simulink model "playback_data_4"  (R2015a)
settings: Solver=FixedStepDiscrete  SolverMode=SingleTasking  StartTime=0  StopTime=time_recorded(end)  FixedStep=sample_time  RelTol=1e-3
undefined symbols (not defined in the file): A1_notch_f1, A2_notch_f1, A_kalman_transverse, A_kalman_vertical, A_lpf_dtau, A_lpf_fourbar_angles, A_lpf_imu, A_lpf_lateral_angle, A_lpf_leg_spring, B1_lpf_dtau, B1_lpf_fourbar_angles, B1_lpf_imu, B1_lpf_lateral_angle, B1_lpf_leg_spring, B1_notch_f1, B2_lpf_dtau, B2_lpf_fourbar_angles, B2_lpf_imu, B2_lpf_lateral_angle, B2_lpf_leg_spring, B2_notch_f1, B_dx_versus_x0, B_kalman_transverse, B_kalman_vertical, backwards_K_front_of_t_row1, backwards_K_front_of_t_row2, backwards_K_sag_of_t, backwards_P_front_of_t, backwards_P_sag_of_t, C_kalman_transverse, C_kalman_vertical, com_leg_motor, com_torso, contact_threshold, control_start_time, d_ankle_to_foot, d_vertical_com, desired_com_forward_velocity, desired_com_lateral_velocity, desired_initial_leg_roll_left, desired_initial_leg_roll_right, desired_lateral_symmetry_angle, desired_standing_torso_pitch, desired_standing_torso_roll, desired_standing_z, desired_torso_pitch, desired_torso_roll, Discrete, fcut_contact, forward_dx_of_dxstar, forward_x_of_dxstar, g, gain_nodes_sea_torque, HIP_MTR_MAX_CONT_TORQUE, HIP_MTR_MAX_TORQUE, i_leg_motor, i_robot, i_torso, initial_dx_estimate, initial_dy_estimate ... (+75)
libraries: simulink x12, ctrlSharedLib x3
(part 4 of 5)

== matlab function playback_data_4/Control/Behavior Control/Primary and Lateral Behavior/Stance/LQR Feedback for Desired Frontal GRF and Roll Accleration ==
  data: hopping input; stance input; GRFy_desired output; ydy input; rolldroll input; symdsym input; zdz input; Fz input; GRF_measured input; ydy_ref input; ddroll_desired output; cost_to_go output double size=1; Roll_star input; symmetry_desired input; K_front input; P_front input; m_torso parameter; m_leg_motor parameter; lateral_offset parameter; com_torso parameter; i_torso parameter; i_leg_motor parameter; k_LQR_frontal_infinite parameter; P_LQR_frontal_infinite parameter; desired_standing_torso_roll parameter; angular_momentum output; frontal_error output
%  x_front = [y, roll, sym, dy, droll, L]; 
function [GRFy_desired, ddroll_desired, cost_to_go, angular_momentum, frontal_error]  =  ...
    LQR_Frontal(hopping, stance, ydy, rolldroll, symdsym, zdz, Fz, GRF_measured,...
           ydy_ref, Roll_star, symmetry_desired, K_front, P_front,...
           m_torso, m_leg_motor, lateral_offset, com_torso, i_torso, i_leg_motor, ...
           k_LQR_frontal_infinite, P_LQR_frontal_infinite, desired_standing_torso_roll)
    
    % Angular momentum about the pelvis in the frontal plane
    d = norm(com_torso(2:3));
    It_f = i_torso(1);
    Im_f = i_leg_motor(1);
    angular_momentum = rolldroll(2)*(m_torso*d^2 + It_f + 2*(m_leg_motor*lateral_offset^2+ Im_f)) -symdsym(2)*(m_leg_motor*lateral_offset^2+Im_f);
    feedforward_Fy = Fz*ydy_ref(1)/zdz(1);
    % feedforward_Fy = Fz*ydy(1)/zdz(1);
    frontal_state = [ydy(1); rolldroll(1); symdsym(1); ydy(2); rolldroll(2); angular_momentum];
    
    if hopping
        frontal_reference = [ydy_ref(1); Roll_star(1); symmetry_desired; ydy_ref(2); Roll_star(2); 0];
        frontal_error = frontal_state - frontal_reference;
        u = [feedforward_Fy;0]-K_front*frontal_error;
        GRFy_desired = u(1);
        ddroll_desired = u(2);
        cost_to_go = 0.5*frontal_error'*P_front*frontal_error;
        GRFy_desired = min(max(GRFy_desired, -0.5*abs(GRF_measured(3))), 0.5*abs(GRF_measured(3))); % saturate to friction cone
    else
        frontal_reference = [ydy_ref(1); desired_standing_torso_roll; symmetry_desired; ydy_ref(2); 0; 0];
        frontal_error = frontal_state - frontal_reference;
        %         frontal_error([1 4]) = 0;
        u = -k_LQR_frontal_infinite*frontal_error;
        %         u = [Fz*ydy(1)/zdz(1); 0]-k_LQR_frontal_infinite*frontal_error;
        GRFy_desired = u(1);
        ddroll_desired = u(2);
        cost_to_go = 0.5*frontal_error'*P_LQR_frontal_infinite*frontal_error;
        GRFy_desired = min(max(GRFy_desired, -0.5*abs(GRF_measured(3))), 0.5*abs(GRF_measured(3)));
    end
    
    if stance == 0
      GRFy_desired = 0;
      ddroll_desired = 0;
      cost_to_go = 0;
    end
end

== matlab function playback_data_4/Control/Behavior Control/Secondary Leg Behavior/Avoid Hitting Mechanical Limits ==
  data: back_cmd output double; front_cmd output double; dback_cmd output double; dfront_cmd output double; ddback_cmd output double; ddfront_cmd output double; back_desired input; dback_desired input; ddback_desired input; front_desired input; dfront_desired input; ddfront_desired input; min_front_bar_angle parameter; max_front_bar_angle parameter; min_back_bar_angle parameter; max_back_bar_angle parameter
%% Avoid joint limits by ensuring we don't command velocities/accelerations that would push us into them when we are close to them.
function [back_cmd, front_cmd, dback_cmd, dfront_cmd, ddback_cmd, ddfront_cmd] ...
    = AvoidFourbarLimits(back_desired,dback_desired, ddback_desired, ...
          front_desired, dfront_desired, ddfront_desired, ...
          min_front_bar_angle, max_front_bar_angle, min_back_bar_angle, max_back_bar_angle)
    [back_cmd, front_cmd, dback_cmd, dfront_cmd, ddback_cmd, ddfront_cmd] = AvoidFourbarLimits(back_desired,dback_desired, ddback_desired, front_desired, dfront_desired, ddfront_desired, min_front_bar_angle, max_front_bar_angle, min_back_bar_angle, max_back_bar_angle);
end

== matlab function playback_data_4/Control/Behavior Control/State Estimation/PositionUsingRobotGeometry ==
  data: right_left input; horizontal_com_position output; roll input; pitch input; yaw input; horizontal_com_velocity output; lateral_com_position output; lateral_com_velocity output; left_leg_sagittal_angle input; left_leg_lateral_angle input; left_leg_length input; right_leg_sagittal_angle input; right_leg_lateral_angle input; right_leg_length input; m_torso parameter; m_leg_motor parameter; m_leg parameter; com_torso parameter; com_leg_motor parameter; lateral_offset parameter; vertical_com_position output; vertical_com_velocity output; com_left_foot output; dcom_left_foot output; com_right_foot output; dcom_right_foot output; com_pelvis output; dcom_pelvis output
% Returns 2D COM relative to primary foot
function [horizontal_com_position, horizontal_com_velocity, ...
          lateral_com_position, lateral_com_velocity, ...
          vertical_com_position, vertical_com_velocity, ...
          com_left_foot, dcom_left_foot, com_right_foot, dcom_right_foot, ....
          com_pelvis, dcom_pelvis] = ...
         ComPositionUsingRobotGeometry(right_left, ...
                                    roll, pitch, yaw, ...
                                    left_leg_sagittal_angle, left_leg_lateral_angle, left_leg_length, ...
                                    right_leg_sagittal_angle, right_leg_lateral_angle, right_leg_length, ...
                                    m_torso, m_leg_motor, m_leg, com_torso, com_leg_motor, lateral_offset)
                    
    q =  [roll(1), pitch(1), yaw(1), left_leg_sagittal_angle(1), left_leg_lateral_angle(1), left_leg_length(1), right_leg_sagittal_angle(1), right_leg_lateral_angle(1), right_leg_length(1)];
    dq = [roll(2), pitch(2), yaw(2), left_leg_sagittal_angle(2), left_leg_lateral_angle(2), left_leg_length(2), right_leg_sagittal_angle(2), right_leg_lateral_angle(2), right_leg_length(2)];
                    
    [ com_pelvis, dcom_pelvis, ...
      com_left_foot, dcom_left_foot, ...
      com_right_foot, dcom_right_foot ] = ...
    ComCalculationFromRobot( q, dq, m_torso, m_leg_motor, m_leg, com_torso, com_leg_motor, lateral_offset );

    if right_left
        com_position = com_right_foot(4:6);
        com_velocity = dcom_right_foot(4:6);
    else
        com_position = com_left_foot(4:6);
        com_velocity = dcom_left_foot(4:6);
    end


    horizontal_com_position = com_position(1);
    horizontal_com_velocity = com_velocity(1);
    lateral_com_position = com_position(2);
    lateral_com_velocity = com_velocity(2);
    vertical_com_position = com_position(3);
    vertical_com_velocity = com_velocity(3);

end

== matlab function playback_data_4/Control/Behavior Control/Torque Distribution Left/Motor Torque Saturation Optimization ==
  data: x1s input; t1 output; x2s input; lambda1 parameter; lambda2 parameter; max_torque_sagittal parameter; t2 output
% Optimal leg motor torque distribution
function [t1, t2] = distribute_torque(x1s, x2s, lambda1, lambda2, max_torque_sagittal)

s = max_torque_sagittal;

% possible solutions
x1 = [                                                      x1s;
                                                            0;
                                                            s;
                                                            0;
                                                           -s;
  (lambda2*s + lambda1*x1s - lambda2*x2s)/(lambda1 + lambda2);
  (lambda1*x1s - lambda2*s + lambda2*x2s)/(lambda1 + lambda2);
  (lambda2*s + lambda1*x1s + lambda2*x2s)/(lambda1 + lambda2);
 -(lambda2*s - lambda1*x1s + lambda2*x2s)/(lambda1 + lambda2)];
 
x2 = [                                                      x2s;
                                                            s;
                                                            0;
                                                           -s;
                                                            0;
  (lambda1*s - lambda1*x1s + lambda2*x2s)/(lambda1 + lambda2);
  (lambda1*s + lambda1*x1s + lambda2*x2s)/(lambda1 + lambda2);
  (lambda1*x1s - lambda1*s + lambda2*x2s)/(lambda1 + lambda2);
 -(lambda1*s + lambda1*x1s - lambda2*x2s)/(lambda1 + lambda2)];

% test constraints
c1 = s - x1 - x2 >= 0;
c2 = s + x1 + x2 >= 0;
c3 = s - x1 + x2 >= 0;
c4 = s + x1 - x2 >= 0;
constraints = c1 & c2 & c3 & c4;

% objective function to maximize
f = -lambda1*(x1-x1s).^2-lambda2*(x2-x2s).^2;
satisfied = find(constraints);
[~,I] = max(f(satisfied));

t1 = x1(satisfied(I));
t2 = x2(satisfied(I));

== matlab function playback_data_4/Control/Behavior Control/State Estimation/Kalman Filtering/eigen values ==
  data: Z input; E output
function E = eigen(Z)
    E = real(eig(Z));
    E = sort(E);
end

== matlab function playback_data_4/Control/Behavior Control/Primary and Lateral Behavior/Flight/Generate Parabolic Foot Trajectories ==
  data: time_remaining input; est_duration input; x_star input; y_star input; x0 input; dx0 input; y0 input; dy0 input; zdz0 input; max_retract input; flight input; z_land parameter; min_f_duration parameter; X_star output size=3; Y_star output size=3; Z_star output size=3
%% Parabolic trajectory generation for x, y, and z
% est_duration: estimated flight time
% time_remaining: time until estimated touchdown
% stance: 1 if in stance, 0 otherwise
% x_star: desired x for foot to COM
% y_star: desired y for foot to COM
% x0: x position at takeoff
% y0: y position at takeoff
% zdz0: [z, dz] at takeoff
% max_retract: how high to lift z for ground clearance
% z_land: nominal z height for landing
% min_f_duration: minimum trajectory time

function [X_star, Y_star, Z_star]  =  ...
          GenerateParabolicFootTrajectory(time_remaining, est_duration,  ...
                               x_star, y_star, x0, dx0, y0, dy0, zdz0, ...
                               max_retract,  flight, z_land, min_f_duration)

if ~flight
    X_star = [0;0;0];
    Y_star = [0;0;0];
    Z_star = [0;0;0];
    return;
end
                           
% we are solving for yawed coordinates xyz of com-foot in flight and
% converting them to joint angles

% estimate z ballistically
% z = z_dz_liftoff(1) + z_dz_liftoff(2)*t_flight -g/2*t_flight^2;
% dz = z_dz_liftoff(2) - g*t_flight;
% 
% z = com_xdx_ydy_zdz(5); dz = com_xdx_ydy_zdz(6);
% time_remaining = (-dz-sqrt(max(dz^2 - 4*g/2*(z_land-z), 0) ) )/ (-g); % ballistic estimate of landing


  % plan a traj from init to desired in estimated duration. Use a
  % discontinuous initial condition if estimated duration too short.
  duration = max(est_duration, min_f_duration);
  t_r = max(min(time_remaining, duration),0);
  % sweep a parabola from x0 to x_star with dx_end = -dx0
  dx_star = dx0;
  x_star_t = x_star + dx_star*t_r + (x0-x_star-dx_star*duration)*(t_r/duration)^2;
  dx_star_t = -dx_star - 2*(x0-x_star-dx_star*duration)*(t_r/duration^2);
  ddx_star_t =  2*(x0-x_star-dx_star*duration)*(1/duration^2);
  
  % same for y
  dy_star = dy0;
  y_star_t = y_star + dy_star*t_r + (y0-y_star-dy_star*duration)*(t_r/duration)^2;
  dy_star_t = -dy_star - 2*(y0-y_star-dy_star*duration)*(t_r/duration^2);
  ddy_star_t =  2*(y0-y_star-dy_star*duration)*(1/duration^2);
  
  % Zero out velocities when out of time
  if time_remaining < 0
    dx_star_t = 0; ddx_star_t = 0;
    dy_star_t = 0; ddy_star_t = 0;
  end 
  
  % split duration into thirds.  First segment: parabola from z0 to
  % max_retract.  Second and third segments, cos to landing.
  z0 = zdz0(1);
  dt3 = duration / 3;
  z_min = z_land - max_retract;
  if t_r > 2*dt3;
    z_star_t = z_min + (z0-z_min)*((t_r-2*dt3)/dt3)^2;
    dz_star_t = -(z0-z_min)*2*(t_r-2*dt3)/dt3/dt3;
    ddz_star_t = (z0-z_min)*2/dt3^2;
  else
    z_star_t = z_land + (z_min-z_land)/2*(1-cos(t_r/(2*dt3)*pi));
    dz_star_t = -(z_min-z_land)/2*sin(t_r/(2*dt3)*pi)*pi/(2*dt3);
    ddz_star_t = (z_min-z_land)/2*cos(t_r/(2*dt3)*pi)*(pi/(2*dt3))^2;
  end
  
  % track a sinusoidal z of amplitude max_retract, finishing a half-cycle by t_end
  X_star = [x_star_t; dx_star_t; ddx_star_t];
  Y_star = [y_star_t; dy_star_t; ddy_star_t];
  Z_star = [z_star_t; dz_star_t; ddz_star_t];

== matlab function playback_data_4/Control/Behavior Control/Primary and Lateral Behavior/Stance/LQR Feedback for Desired Vertical GRF ==
  data: hopping input; stance input; zdzddz_ref input size=3; GRFz_desired output; z_state input; leg_length input; k_LQR_vertical parameter; P_LQR_vertical parameter; k_vertical_winch parameter; m_total_real parameter; g parameter; cost_to_go output double size=1; max_leg_length parameter
%% LQR for z during stance

% stance: 1 if in stance, 0 otherwise
% z_state: [z, dz] current estimate
% zdzddz_ref: reference trajectory for z position, velocity, and acceleration


% GRFz_desired: desired z GRF
% cost_to_go: remaining LQR cost

function [GRFz_desired, cost_to_go]   =  ...
               LQR_Vertical_Height(hopping, stance, zdzddz_ref, z_state, leg_length,...
                                   k_LQR_vertical, P_LQR_vertical, k_vertical_winch, m_total_real, g, max_leg_length)

    z_ref = zdzddz_ref(1:2);     
    ddz_ref = zdzddz_ref(3);
    z_error = (z_state - z_ref);
    GRFz_desired = m_total_real*(g+ddz_ref) - k_LQR_vertical*z_error;
    
    if z_ref(2) < 0
        GRFz_desired = max(50, GRFz_desired);
    elseif leg_length(1) >= max_leg_length
        GRFz_desired = 0;
    end
    
    if ~hopping
        GRFz_desired = m_total_real*g - k_vertical_winch*z_error;
        GRFz_desired = max(200, GRFz_desired);
    end
    
    cost_to_go = z_error'*P_LQR_vertical*z_error;
    
    if stance == 0
      GRFz_desired = 0;
      cost_to_go = 0;
    end
end

== matlab function playback_data_4/Control/Behavior Control/Primary and Lateral Behavior/Circular Buffer/Buffer6 ==
  data: data input; buffer output size=recorded_steps; trigger input; buffer_size input
function buffer  = buffer_data(data, trigger, buffer_size)

    persistent buffer_memory
    coder.varsize('buffer_memory',100);
    if isempty(buffer_memory)
        buffer_memory = [];
    end
    
    if trigger
        buffer_memory = [data; buffer_memory];
        if size(buffer_memory, 1) > buffer_size
            buffer_memory = buffer_memory(1:buffer_size,:);
        end
    end
    
    buffer = buffer_memory;

end

== matlab function playback_data_4/Control/Behavior Control/Primary and Lateral Behavior/Stance/COM X,Y,Z  trajectory generation ==
  data: stance input; hopping input; x_0 output size=1; y_0 output size=1; z_ref output size=1; dz_ref output size=1; ddz_ref output size=1; x_ref output size=1; dx_ref output size=1; y_ref output size=1; dy_ref output size=1; t input size=1; dx0 input; dy0 input; target_DX input; target_DY input; z_rest_new parameter; z_amplitude parameter; spring_frequency parameter; phase_0 parameter; forward_x_of_dxstar parameter; forward_dx_of_dxstar parameter; target_dx_range parameter; T_s parameter; desired_standing_z parameter
%% COM trajectory generation for stance & foot placement for flight

% Outputs:
% x_0: desired x position for COM at touchdown
% y_0: desired y position for COM at touchdown
% [z_ref, dz_ref, ddz_ref]: reference trajectory for vertical
% [x_ref, dx_ref]: reference trajectory for forward
% [y_ref, dy_ref]: reference trajectory for lateral

% Inputs:
% t: time since touchdown
% dx0: touchdown x velocity
% dy0: touchdown y velocity
% target_DX: desired x velocity at takeoff
% s_duration: nominal stance time
% z_rest_new: z height of oscillation
% target_dx_range: full range of possible x velocities in lookup table
% forward_x_of_dxstar: master lookup table for x trajectories
% T_s: tabled vector from 0 to s_duration

function [x_0, y_0,...
          z_ref, dz_ref, ddz_ref, ...
          x_ref, dx_ref, y_ref, dy_ref] ...
          = ReferenceTrajectory(stance, hopping, t, dx0, dy0, target_DX, target_DY, z_rest_new, z_amplitude, ...
            spring_frequency, phase_0, forward_x_of_dxstar, forward_dx_of_dxstar, ...
            target_dx_range, T_s,...
            desired_standing_z)
        
    % Z trajectory 
    z_ref =  z_rest_new + z_amplitude*sin(spring_frequency*t+phase_0);
    dz_ref = z_amplitude*spring_frequency*cos(spring_frequency*t+phase_0);
    ddz_ref = -z_amplitude*spring_frequency^2*sin(spring_frequency*t+phase_0);
    
    % saturate t and initial velocity to reference library
    t_sat = max( min(t, T_s(end)), 0);

    % [X, dX] trajectory from 0 to s_duration
    forward_x_given_dxstar = squeeze(interp1(target_dx_range, forward_x_of_dxstar, target_DX));
    forward_dx_given_dxstar = squeeze(interp1(target_dx_range, forward_dx_of_dxstar, target_DX));

    dx0 = max( min(dx0, max(forward_dx_given_dxstar(:,1))), min(forward_dx_given_dxstar(:,1)) );
    x_ref  = interp2(T_s, forward_dx_given_dxstar(:,1), forward_x_given_dxstar, t_sat, dx0);
    dx_ref = interp2(T_s, forward_dx_given_dxstar(:,1), forward_dx_given_dxstar, t_sat, dx0);
    x_0 = interp1(forward_dx_given_dxstar(:,1), forward_x_given_dxstar(:,1), dx0);

    % [Y, dY] trajectory from 0 to s_duration
    % Y uses same library as X
    forward_y_given_dxstar = squeeze(interp1(target_dx_range, forward_x_of_dxstar, target_DY));
    forward_dy_given_dxstar = squeeze(interp1(target_dx_range, forward_dx_of_dxstar, target_DY));

    dy0 = max( min(dy0, max(forward_dy_given_dxstar(:,1))), min(forward_dy_given_dxstar(:,1)) );
    y_ref  = interp2(T_s, forward_dy_given_dxstar(:,1), forward_y_given_dxstar, t_sat, dy0);
    dy_ref = interp2(T_s, forward_dy_given_dxstar(:,1), forward_dy_given_dxstar, t_sat, dy0);
    y_0 = interp1(forward_dy_given_dxstar(:,1), forward_y_given_dxstar(:,1), dy0);
    
    if ~hopping % Standing
        z_ref = desired_standing_z;
        dz_ref = 0;
        ddz_ref = 0;
        x_ref = 0;
        dx_ref = 0;
        y_ref = 0;
        dy_ref =0;
    elseif ~stance % Flight
        z_ref = 0;
        dz_ref = 0;
        ddz_ref = 0;
        x_ref = 0;
        dx_ref = 0;
        y_ref = 0;
        dy_ref =0;    
    end
  
end

== matlab function playback_data_4/Control/Behavior Control/Primary and Lateral Behavior/Stance/Lookup finite horizon LQR gain ==
  data: K_sag output size=[1,4]; P_sag output size=[4,4]; t_forward input; backwards_K_sag_of_t parameter; backwards_K_front_of_t_row1 parameter; backwards_K_front_of_t_row2 parameter; T_lqr parameter; stance_duration parameter; K_front output size=[2,6]; backwards_P_sag_of_t parameter; P_front output size=[6,6]; backwards_P_front_of_t parameter
%% Interpolates pregenerated finite horizon LQR gain tables 
% sagittal_state: [X, Pitch, dX, dPtich]
% frontal state: [Y; Roll; sym; dY; dRoll; angular_momentum];
function [K_sag, P_sag, K_front, P_front]  =  FiniteHorizonLQRLookup(t_forward, backwards_K_sag_of_t, backwards_K_front_of_t_row1, backwards_K_front_of_t_row2, T_lqr, stance_duration, backwards_P_sag_of_t, backwards_P_front_of_t)
  t = stance_duration - t_forward; % gains are scheduled w.r.t time until end.                                     
  t = min(max(t, min(T_lqr)), max(T_lqr));
  K_sag = interp1(T_lqr, backwards_K_sag_of_t, t);
  P_sag = squeeze(interp1(T_lqr,backwards_P_sag_of_t,t));

  % inputs for frontal LQR: backwards_K_front_of_t_row1, backwards_K_front_of_t_row2
  K_front_row1 = interp1(T_lqr, backwards_K_front_of_t_row1, t);
  K_front_row2 = interp1(T_lqr, backwards_K_front_of_t_row2, t);
  K_front = [K_front_row1; K_front_row2];
  P_front = squeeze(interp1(T_lqr,backwards_P_front_of_t,t));
end

== matlab function playback_data_4/Control/Behavior Control/Primary and Lateral Behavior/Flight/Convert COM Position to Joint Angles + Leg Length  ==
  data: hopping input; desired_leg_length output; X_star input; Y_star input; Z_star input; right_left input; com_pelvis_body input; desired_alpha output; desired_beta output; dcom_pelvis_body input; roll input; pitch input; sagittal_angle input; lateral_angle input; leg_length input; lateral_offset parameter; desired_initial_leg_roll_right parameter; desired_initial_leg_roll_left parameter; d_vertical_com parameter; desired_standing_z parameter
function [ desired_leg_length, desired_alpha, desired_beta ]  =  ...
          ConvertToJointAnglesAndLegLength(hopping, X_star, Y_star, Z_star, right_left,...
                           com_pelvis_body, dcom_pelvis_body, ...
                           roll, pitch, sagittal_angle, lateral_angle, leg_length,...
                           lateral_offset, desired_initial_leg_roll_right, desired_initial_leg_roll_left, d_vertical_com, desired_standing_z) 

    q = [roll(1), pitch(1), sagittal_angle(1), lateral_angle(1), leg_length(1)];
    dq = [roll(2), pitch(2), sagittal_angle(2), lateral_angle(2), leg_length(2)];
    [desired_alpha, desired_beta, desired_leg_length]  =  ConvertComPositionToLegAnglesAndLegLength(X_star, Y_star, Z_star, right_left, com_pelvis_body, dcom_pelvis_body, q, dq, lateral_offset);   
                       
    if ~hopping
        desired_leg_length = [desired_standing_z-d_vertical_com; 0; 0];
        desired_alpha = [pi; 0; 0];
        desired_beta = [desired_initial_leg_roll_left; 0; 0];
        if right_left
            desired_beta = [desired_initial_leg_roll_right; 0; 0];
        end
    end
    
end

== matlab function playback_data_4/Control/Behavior Control/Primary and Lateral Behavior/Circular Buffer/Buffer7 ==
  data: data input; buffer output size=recorded_steps; trigger input; buffer_size input
function buffer  = buffer_data(data, trigger, buffer_size)

    persistent buffer_memory
    coder.varsize('buffer_memory',100);
    if isempty(buffer_memory)
        buffer_memory = [];
    end
    
    if trigger
        buffer_memory = [data; buffer_memory];
        if size(buffer_memory, 1) > buffer_size
            buffer_memory = buffer_memory(1:buffer_size,:);
        end
    end
    
    buffer = buffer_memory;

end

== matlab function playback_data_4/Control/Behavior Control/Secondary Leg Behavior/Virtual Leg to Four Bar ==
  data: l_leg input; dl_leg input; ddl_leg input; phi input; dphi input; ddphi input; back output; dback output; ddback output; front output; dfront output; ddfront output
function [back, dback, ddback, front, dfront, ddfront] = VirtualLegToFourBar(l_leg, dl_leg, ddl_leg, phi, dphi, ddphi)
    [back, dback, ddback, front, dfront, ddfront] = VirtualLegToFourBar(l_leg, dl_leg, ddl_leg, phi, dphi, ddphi);
end

== matlab function playback_data_4/Control/Behavior Control/Primary and Lateral Behavior/Closed Loop Compensation/CLOSED LOOP COMPENSATION X FOR VAIRABLE SPEED ==
  data: A_cl input; epsilon input; c input; delta_s_i input; dx_star input; B_cl input; delta_ux output
function delta_ux  = closed_loop_compensation_dxstar...
         (A_cl,epsilon, c, delta_s_i, dx_star, B_cl)
% assume form of delta_s_{i+1} = A_cl*delta_s_i + epsilon +c*dx_star + B_cl*delta_ux
% where delta measures deviation from deadbeat case. solve for
% delta_ux = (-A_cl*delta_s_i-epsilon - c*dxstar)/B_cl to achieve deadbeat
delta_ux = (-A_cl*delta_s_i - epsilon - c*dx_star)/B_cl;

== matlab function playback_data_4/Control/Behavior Control/Primary and Lateral Behavior/Closed Loop Compensation/ESTIMATE CLOSED LOOP ERROR X FOR VARIABLE SPEED ==
  data: dx_land_hist input; A_cl output; delta_ux_hist input; dx_lift_hist input; dx_star_hist input; B_dx_versus_x0 parameter; W_real input; epsilon_0 output; c output; A_cl_nb output; epsilon_0_nb output; c_nb output
function [A_cl, epsilon_0, c, ...
          A_cl_nb, epsilon_0_nb, c_nb] = error_fitting_dxstar...
         (dx_land_hist, delta_ux_hist, dx_lift_hist, dx_star_hist,...
          B_dx_versus_x0, W_real)
% data_length = min([length(dx_lift_hist), filter_length]);
data_length = length(dx_lift_hist);
assert(data_length < 100);
% add fake data
fake_dx_land_err_magnitude = 0.1; fake_dx_star_magnitude = 0.1;
[fgrid_dx_land_err, fgrid_dx_star, fgrid_dx_lift_err] = ...
    meshgrid(fake_dx_land_err_magnitude*[-1 1],fake_dx_star_magnitude*[-1 1],0);
fake_data_length = numel(fgrid_dx_land_err);
fake_dx_land_err = fgrid_dx_land_err(:);
fake_dx_star = fgrid_dx_star(:);
fake_dx_lift_err = fgrid_dx_lift_err(:);
fake_delta_ux = zeros(fake_data_length,1);
% assert(fake_data_length<100);
% assert(filter_length<100);
% fake_dx_land_err = linspace(-0.1, 0.1, fake_data_length)';
% fake_dx_lift_err = zeros(fake_data_length,1);
% fake_delta_ux = zeros(fake_data_length,1);
% fake_dx_star = linspace(-0.25, 0.25, fake_data_length)';
dx_land_err = [reshape(dx_land_hist(1:data_length)-dx_star_hist(1:data_length),...
                       data_length, 1); fake_dx_land_err];
dx_lift_err = [reshape(dx_lift_hist(1:data_length)-dx_star_hist(1:data_length),...
                       data_length, 1); fake_dx_lift_err];
dx_star = [reshape(dx_star_hist(1:data_length), data_length,1); fake_dx_star];
delta_ux = [reshape(delta_ux_hist(1:data_length), data_length, 1); fake_delta_ux];
% weighted least squares
W = diag([W_real*ones(1,data_length), ones(1,fake_data_length)]);
Y = dx_lift_err - B_dx_versus_x0*delta_ux;
X = [dx_land_err, dx_star, ones(data_length+fake_data_length,1)];
% linear regression for s_{i+1}-s0 = A_cl*(s_i-s0) + epsilon_0 + c(s0) + B*delta_u
% solve for Y = X*beta, beta column vector
beta_hat = (X'*W*X)\X'*W*Y;
W_nobias = diag([W_real*ones(1,data_length), 0.001*ones(1,fake_data_length)]);
beta_hat_nobias = (X'*W_nobias*X)\X'*W_nobias*Y;
A_cl = beta_hat(1);
c = beta_hat(2);
epsilon_0 = beta_hat(3);
A_cl_nb = beta_hat_nobias(1);
c_nb = beta_hat_nobias(2);
epsilon_0_nb = beta_hat_nobias(3);

== matlab function playback_data_4/Control/Behavior Control/Primary and Lateral Behavior/Closed Loop Compensation/CLOSED LOOP COMPENSATION Y FOR VAIRABLE SPEED ==
  data: A_cl input; epsilon input; c input; delta_s_i input; dx_star input; B_cl input; delta_ux output
function delta_ux  = closed_loop_compensation_dxstar...
         (A_cl,epsilon, c, delta_s_i, dx_star, B_cl)
% assume form of delta_s_{i+1} = A_cl*delta_s_i + epsilon +c*dx_star + B_cl*delta_ux
% where delta measures deviation from deadbeat case. solve for
% delta_ux = (-A_cl*delta_s_i-epsilon - c*dxstar)/B_cl to achieve deadbeat
delta_ux = (-A_cl*delta_s_i - epsilon - c*dx_star)/B_cl;

== matlab function playback_data_4/Control/Behavior Control/Primary Secondary Leg Swap/ToggleRightLeftLeg ==
  data: toggle input boolean; right_left output double; previous_right_left input double
function right_left = ToggleRightLeftLeg(toggle, previous_right_left)
    
    if toggle
        right_left = -previous_right_left + 1;
    else
        right_left = previous_right_left;
    end

end

== matlab function playback_data_4/Control/Behavior Control/Primary and Lateral Behavior/Desired Forward Velocity ==
  data: dx_takeoff input; desired_dx output; desired_forward_velocity input; forward_velocity_target_step parameter
function desired_dx = dx_command(dx_takeoff, desired_forward_velocity, forward_velocity_target_step)
    desired_direction = sign(desired_forward_velocity);
    desired_dx = dx_takeoff + desired_direction*forward_velocity_target_step;
    desired_dx = max(min(desired_dx, abs(desired_forward_velocity)),-abs(desired_forward_velocity));
end

== matlab function playback_data_4/Control/Behavior Control/Force Estimation/3D Forward Dynamics yawed ==
  data: right_or_left input; torso_roll input size=2; torso_pitch input double size=2; torso_yaw input double size=2; primary_sagittal_leg_angle input double size=2; primary_leg_length input double size=2; primary_leg_roll input double size=2; secondary_leg_roll input double size=2; primary_leg_torque input; primary_leg_force input; primary_lateral_torque input; secondary_lateral_torque input; R_GRF output double size=3; L_GRF output size=3; ddroll output double; g parameter; m_leg_motor parameter; m_torso parameter; i_torso parameter; i_leg_motor parameter; lateral_offset parameter; com_torso parameter; torso_centerline_roll_offset_angle parameter
%% Forward 3D ATRIAS dynamics
function [R_GRF, L_GRF, ddroll]  =  ForwardDynamics3D(right_or_left, ...
                                                      torso_roll, torso_pitch, torso_yaw, ...
                                                      primary_sagittal_leg_angle, primary_leg_length,...
                                                      primary_leg_roll, secondary_leg_roll, ...
                                                      primary_leg_torque, primary_leg_force, ...
                                                      primary_lateral_torque, secondary_lateral_torque, ...
                                                      g, m_leg_motor, m_torso, i_torso, i_leg_motor, lateral_offset, com_torso, torso_centerline_roll_offset_angle)

    d = norm(com_torso(2:3));
    It = mean(i_torso);
    Im = mean(i_leg_motor);
    
    phi    = torso_roll(1) + torso_centerline_roll_offset_angle;  % roll
    theta  = torso_pitch(1);                   % pitch
    alpha1 = primary_sagittal_leg_angle(1);    % primary sagittal leg angle
    beta1  = primary_leg_roll(1);              % primary leg roll
    beta2  = secondary_leg_roll(1);            % secondary leg roll
    if right_or_left
        beta1 = beta1 - torso_centerline_roll_offset_angle;
        beta2 = beta2 + torso_centerline_roll_offset_angle;
    else
        beta1 = beta1 + torso_centerline_roll_offset_angle;
        beta2 = beta2 - torso_centerline_roll_offset_angle;
    end 
    l1     = primary_leg_length(1);            % primary leg length
    
    dphi    = torso_roll(2);
    dtheta  = torso_pitch(2);
    dpsi    = torso_yaw(2);
    dalpha1 = primary_sagittal_leg_angle(2);
    dbeta1  = primary_leg_roll(2);
    dbeta2  = secondary_leg_roll(2);
    dl1     = primary_leg_length(2);
    
    
    tau_a1 = primary_leg_torque;
    tau_b1 = primary_lateral_torque;
    tau_b2 = secondary_lateral_torque;
    F_l1 = primary_leg_force;

    if right_or_left == 1
      A = A_fwd_yawed_right(lateral_offset,d,m_leg_motor,m_torso,It,Im,phi,theta,alpha1,beta1,beta2,l1);
      B = B_fwd_yawed_right(lateral_offset,d,g,m_leg_motor,m_torso,It,Im,phi,theta,alpha1,beta1,beta2,l1,dphi,dtheta,dpsi,dalpha1,dbeta1,dbeta2,dl1,tau_a1,tau_b1,tau_b2,F_l1);
    else
      A = A_fwd_yawed_left(lateral_offset,d,m_leg_motor,m_torso,It,Im,phi,theta,alpha1,beta1,beta2,l1);
      B = B_fwd_yawed_left(lateral_offset,d,g,m_leg_motor,m_torso,It,Im,phi,theta,alpha1,beta1,beta2,l1,dphi,dtheta,dpsi,dalpha1,dbeta1,dbeta2,dl1,tau_a1,tau_b1,tau_b2,F_l1);
    end
    
    x_fwd = A \ B;
    ddroll = x_fwd(4);
    GRF = zeros(3,1);
    GRF(1) = x_fwd(11);
    GRF(2) = x_fwd(12);
    GRF(3) = x_fwd(13); 
    
    if right_or_left == 1
        R_GRF = GRF;
        L_GRF = [0;0;0];
    else
        R_GRF = [0;0;0];
        L_GRF = GRF;
    end
end

== matlab function playback_data_4/Control/Behavior Control/Primary and Lateral Behavior/Flight/Avoid Hitting Mechanical Limits ==
  data: back_cmd output double; front_cmd output double; dback_cmd output double; dfront_cmd output double; ddback_cmd output double; ddfront_cmd output double; back_desired input; dback_desired input; ddback_desired input; front_desired input; dfront_desired input; ddfront_desired input; min_front_bar_angle parameter; max_front_bar_angle parameter; min_back_bar_angle parameter; max_back_bar_angle parameter
%% Avoid joint limits by ensuring we don't command velocities/accelerations that would push us into them when we are close to them.
function [back_cmd, front_cmd, dback_cmd, dfront_cmd, ddback_cmd, ddfront_cmd] ...
    = AvoidFourbarLimits(back_desired,dback_desired, ddback_desired, ...
          front_desired, dfront_desired, ddfront_desired, ...
          min_front_bar_angle, max_front_bar_angle, min_back_bar_angle, max_back_bar_angle)
    [back_cmd, front_cmd, dback_cmd, dfront_cmd, ddback_cmd, ddfront_cmd] = AvoidFourbarLimits(back_desired,dback_desired, ddback_desired, front_desired, dfront_desired, ddfront_desired, min_front_bar_angle, max_front_bar_angle, min_back_bar_angle, max_back_bar_angle);
end

== matlab function playback_data_4/Control/Behavior Control/Primary and Lateral Behavior/Flight/Virtual Leg to Four Bar ==
  data: l_leg input; dl_leg input; ddl_leg input; phi input; dphi input; ddphi input; back output; dback output; ddback output; front output; dfront output; ddfront output
function [back, dback, ddback, front, dfront, ddfront] = VirtualLegToFourBar(l_leg, dl_leg, ddl_leg, phi, dphi, ddphi)
    [back, dback, ddback, front, dfront, ddfront] = VirtualLegToFourBar(l_leg, dl_leg, ddl_leg, phi, dphi, ddphi);
end

== matlab function playback_data_4/Control/Behavior Control/Primary and Lateral Behavior/Flight/Lateral Flight Control ==
  data: hopping input; tau_primary output; tau_secondary output; RightLeftPrimary input; TorsoRoll input; LLegRoll input; RLegRoll input; Beta1_star input; Roll_star input; K_right_lat_flight parameter; K_left_lat_flight parameter; K_right_lat_flight_winch parameter; K_left_lat_flight_winch parameter; Q_phibeta1beta2 parameter; Q_phibeta1beta2_winch parameter; m_torso parameter; m_leg_motor parameter; com_torso parameter; i_torso parameter; i_leg_motor parameter; g parameter; lateral_offset parameter; adjusted_ref output; feedforward output; desired_initial_leg_roll_left parameter; desired_initial_leg_roll_right parameter
% full_state = [Roll; Beta1; Beta2; dRoll; dBeta1; dBeta2];
function [tau_primary, tau_secondary, ...
          adjusted_ref, feedforward] = lateral_flight_control(hopping, RightLeftPrimary,...
          TorsoRoll, LLegRoll, RLegRoll, Beta1_star, Roll_star,...
          K_right_lat_flight, K_left_lat_flight, K_right_lat_flight_winch, K_left_lat_flight_winch, Q_phibeta1beta2, Q_phibeta1beta2_winch,...
          m_torso, m_leg_motor, com_torso, i_torso, i_leg_motor, g, lateral_offset, desired_initial_leg_roll_left, desired_initial_leg_roll_right)

    d = norm(com_torso(2:3));
    It_f = i_torso(1);
    Im_f = i_leg_motor(1); 
    phidphi = TorsoRoll; 
    symdsym = LLegRoll-RLegRoll;
    ang_mom = phidphi(2)*(m_torso*d^2 + It_f + 2*(m_leg_motor*lateral_offset^2+ Im_f)) -symdsym(2)*(m_leg_motor*lateral_offset^2+Im_f);

    if RightLeftPrimary == 1
        Beta1 = RLegRoll;
        Beta2 = LLegRoll;
        Beta2_star = [desired_initial_leg_roll_left; 0; 0];
    else
        Beta1 = LLegRoll;
        Beta2 = RLegRoll;
        Beta2_star = [desired_initial_leg_roll_right; 0; 0];
    end    
    
    if ~hopping
        Q_phibeta1beta2 = Q_phibeta1beta2_winch;
        K_right_lat_flight = K_right_lat_flight_winch;
        K_left_lat_flight = K_left_lat_flight_winch;
    end

    ref_old = [Roll_star(1); Beta1_star(1); Beta2_star(1)];
    dref_old = [0; Beta1_star(2); Beta2_star(2)];
    ddref_old = [0; Beta1_star(3); Beta2_star(3)];
    
    % eliminate beta2 from state using momentum:
    % s_old = T*s_new+D(t); s_new = [phi; beta1];
    % dbeta_R = L/(Im_f+mm*r^2) - (It_f+mm*d^2+2*Im_f+2*mm*r^2)/(Im_f+mm*r^2)*dphi + dbeta_L 
    % beta_R = beta_R0 + L/(Im_f+mm*r^2)*t - ((It_f+mm*d^2+2*Im_f+2*mm*r^2)/(Im_f+mm*r^2)*(phi-phi0) + (beta_L-beta_L0)
    % beta_R = [beta_R0-b1*phi0-b2*beta_L0 + a*t + b1*phi + b2*beta_L;
    
    if RightLeftPrimary == 1 % beta_2 is beta_L, beta_1 is beta_R, eliminate beta2
      a = -ang_mom/(Im_f+m_leg_motor*lateral_offset^2);
      b1 = (It_f+m_torso*d^2+2*Im_f+2*m_leg_motor*lateral_offset^2)/(Im_f+m_leg_motor*lateral_offset^2); b2 = 1;
    else
      a = +ang_mom/(Im_f+m_leg_motor*lateral_offset^2);
      b1 = -(It_f+m_torso*d^2+2*Im_f+2*m_leg_motor*lateral_offset^2)/(Im_f+m_leg_motor*lateral_offset^2); b2 = 1;
    end
    
    T = [eye(2); b1, b2];
    %  D = [0; 0; 0; 0; beta_R0 - b1*phi0 - b2*beta_L0 + a*t; a];
    D = [0;0; Beta2(1) - b1*phidphi(1) - b2*Beta1(1)];
    
    % old cost (state s)  (s-s_ref)' * Q *(s-s_ref);
    % new cost (state r) =(T*r+D-s_ref)'*Q*(T*r+D-s_ref);
    %                    =(r+ (T'QT)^{-1}T'Q(D-s_ref))'*T'QT*
    %                     (r + (T'QT)^{-1}T'Q(D-s_ref))
    
    
    Q_new = T'*Q_phibeta1beta2*T;
    ref_new = Q_new\T'*Q_phibeta1beta2*(ref_old-D);
    ref_new_vel = Q_new\T'*Q_phibeta1beta2*(dref_old - [0;0; a]);
    ref_accels = Q_new\T'*Q_phibeta1beta2*(ddref_old);

    % A_phidphi_betadbeta1 = [0 1 0 0; 0 0 0 0; 0 0 0 1; 0 0 0 0];
    % assume beta1 is right
    if RightLeftPrimary == 1
        B_new_state = [0 0; 0 0; -1/(It_f+m_torso*d^2), 1/(It_f+m_torso*d^2); 1/(It_f+m_torso*d^2)+1/(Im_f+m_leg_motor*lateral_offset^2), -1/(It_f+m_torso*d^2)];
    else
        B_new_state = [0 0; 0 0; 1/(It_f+m_torso*d^2), -1/(It_f+m_torso*d^2); 1/(It_f+m_torso*d^2)+1/(Im_f+m_leg_motor*lateral_offset^2), -1/(It_f+m_torso*d^2)];
    end      
    
    %   K = lqr(A_phidphi_betadbeta1, B_phidphi_betadbeta1, Q_new, R_lat_flight);
    if RightLeftPrimary == 1
      K = K_right_lat_flight;
    else
      K = K_left_lat_flight;
    end

    new_state = [phidphi(1); Beta1(1); phidphi(2); Beta1(2)];
    new_ref_traj = [ref_new; ref_new_vel];

    feedforward = B_new_state([3 4],:)\ref_accels;
    if ~hopping, feedforward = -(m_leg_motor)*g*lateral_offset*ones(2,1); end
    tau_lqr = feedforward - K*(new_state-new_ref_traj);
    tau_1 = tau_lqr(1); tau_2 = tau_lqr(2);
    implied_beta2_star = [0 0 1]*(T*ref_new+D);
    implied_dbeta2_star = [0 0 1]*(T*ref_new_vel+[0; 0; a]);
    % implied_betadbeta2_star = [0 0 0 0 1 0; 0 0 0 0 0 1]*(T*ref_new+D);
    adjusted_ref = [ref_new; implied_beta2_star; ref_new_vel; implied_dbeta2_star];

    tau_primary = tau_1;
    tau_secondary = tau_2;

== matlab function playback_data_4/Control/Behavior Control/Primary and Lateral Behavior/ToggleRightLeftLeg ==
  data: toggle input boolean; direction output double; previous input double
function direction = TogglePositiveNegative(toggle, previous)
    
    if toggle
        direction = -previous;
    else
        direction = previous;
    end

end

== matlab function playback_data_4/Control/Behavior Control/Secondary Leg Behavior/Mirrored Leg Length Target ==
  data: primary_l_leg input; l_leg output; dl_leg output; primary_dl_leg input; l_retract_swing_min parameter; l_retract_swing_max parameter; ddl_leg output; l_retract_delta parameter
function [l_leg, dl_leg, ddl_leg] = LegLengthTarget(primary_l_leg, primary_dl_leg, l_retract_swing_min, l_retract_swing_max, l_retract_delta)

    l_leg = primary_l_leg - l_retract_delta;
    dl_leg = 0;
    ddl_leg = 0;
    if l_leg > l_retract_swing_min && l_leg < l_retract_swing_max
        dl_leg = primary_dl_leg;
    else
        l_leg = max(min(l_leg, l_retract_swing_max), l_retract_swing_min);
    end

end

== matlab function playback_data_4/Control/Behavior Control/Secondary Leg Behavior/Back//Front Motor PD/Motor Efficiency ==
  data: rpm input; mu output; load_torque input
function mu = HarmonicDriveEfficiency(rpm, load_torque)
    mu = HarmonicDriveEfficiency(rpm, load_torque);
end

== matlab function playback_data_4/Control/Behavior Control/Primary and Lateral Behavior/Stance/3D Inverse Dynamics yawed ==
  data: right_or_left input; primary_leg_torque output double size=1; torso_roll input double size=2; torso_pitch input double size=2; torso_yaw input size=2; primary_sagittal_leg_angle input size=2; primary_leg_length input size=2; primary_leg_roll input size=2; secondary_leg_roll input size=2; GRF_desired input double size=3; ddRoll_desired input double size=1; g parameter; primary_lateral_torque output double size=1; secondary_lateral_torque output double size=1; primary_leg_force output double size=1; m_leg_motor parameter; m_torso parameter; i_torso parameter; i_leg_motor parameter; lateral_offset parameter; com_torso parameter; torso_centerline_roll_offset_angle parameter
%% Inverse dynamics
function [primary_leg_torque, primary_lateral_torque, secondary_lateral_torque, primary_leg_force]  =  InverseDynamics3D(right_or_left,...
                                                                                                                         torso_roll, torso_pitch, torso_yaw, ...
                                                                                                                         primary_sagittal_leg_angle, primary_leg_length, ...
                                                                                                                         primary_leg_roll, secondary_leg_roll, ...
                                                                                                                         GRF_desired, ddRoll_desired, ...
                                                                                                                         g, m_leg_motor, m_torso, i_torso, i_leg_motor, lateral_offset, com_torso, torso_centerline_roll_offset_angle)

    d = norm(com_torso(2:3));
    It = mean(i_torso);
    Im = mean(i_leg_motor);
    
    phi    = torso_roll(1) + torso_centerline_roll_offset_angle; % roll
    theta  = torso_pitch(1);                   % pitch
    alpha1 = primary_sagittal_leg_angle(1);    % primary sagittal leg angle
    beta1  = primary_leg_roll(1);              % primary leg roll
    beta2  = secondary_leg_roll(1);            % secondary leg roll
    if right_or_left
        beta1 = beta1 - torso_centerline_roll_offset_angle;
        beta2 = beta2 + torso_centerline_roll_offset_angle;
    else
        beta1 = beta1 + torso_centerline_roll_offset_angle;
        beta2 = beta2 - torso_centerline_roll_offset_angle;
    end 
    l1     = primary_leg_length(1);            % primary leg length
    
    dphi    = torso_roll(2);
    dtheta  = torso_pitch(2);
    dpsi    = torso_yaw(2);
    dalpha1 = primary_sagittal_leg_angle(2);
    dbeta1  = primary_leg_roll(2);
    dbeta2  = secondary_leg_roll(2);
    dl1     = primary_leg_length(2);

    Fx = GRF_desired(1);
    Fy = GRF_desired(2);
    Fz = GRF_desired(3);
    ddphi = ddRoll_desired;

    if right_or_left == 1
      A = A_id_roll_yawed_right(lateral_offset,d,m_leg_motor,m_torso,It,Im,phi,theta,alpha1,beta1,beta2,l1);     
      B = B_id_roll_yawed_right(lateral_offset,d,g,m_leg_motor,m_torso,It,Im,phi,theta,alpha1,beta1,beta2,l1,dphi,dtheta,dpsi,dalpha1,dbeta1,dbeta2,dl1,Fx,Fy,Fz,ddphi);
    else
      A = A_id_roll_yawed_left(lateral_offset,d,m_leg_motor,m_torso,It,Im,phi,theta,alpha1,beta1,beta2,l1);     
      B = B_id_roll_yawed_left(lateral_offset,d,g,m_leg_motor,m_torso,It,Im,phi,theta,alpha1,beta1,beta2,l1,dphi,dtheta,dpsi,dalpha1,dbeta1,dbeta2,dl1,Fx,Fy,Fz,ddphi);
    end        
    
    x_id_roll = A \ B;
    primary_leg_torque = x_id_roll(10);
    primary_lateral_torque = x_id_roll(11);
    secondary_lateral_torque = x_id_roll(12);
    primary_leg_force = x_id_roll(13);
end

== matlab function playback_data_4/Control/Behavior Control/Force Estimation/Leg Force Measurements/SeaTorques1 ==
  data: deflections input; tau output; k_sea_high parameter
function tau = SeaSpringForce(deflections, k_sea_high)
    tau = SeaSpringForce(deflections, k_sea_high);
end

== matlab function playback_data_4/Control/Behavior Control/Primary and Lateral Behavior/Flight/Avoid Virtual Leg Length Limits ==
  data: l_leg_desired input; dl_leg_desired input; ddl_leg_desired input; l_leg_cmd output double; dl_leg_cmd output double; ddl_leg_cmd output double; min_leg_length parameter; max_leg_length parameter
%% Avoid virtual leg length limits by ensuring we don't command position/velocities/accelerations that would hit them.
function [l_leg_cmd, dl_leg_cmd, ddl_leg_cmd] = AvoidVirtualLengthLimits(l_leg_desired, dl_leg_desired, ddl_leg_desired, min_leg_length, max_leg_length)
    [l_leg_cmd, dl_leg_cmd, ddl_leg_cmd] = AvoidVirtualLengthLimits(l_leg_desired, dl_leg_desired, ddl_leg_desired, min_leg_length, max_leg_length);
end

== matlab function playback_data_4/Control/Behavior Control/Primary and Lateral Behavior/Flight/Calculate Time Until Touchdown ==
  data: z_dz input; t output; z_land parameter; g parameter
function t = EstimateTouchdown(z_dz, z_land, g)
  z_hat = z_dz(1); 
  dz_hat = z_dz(2);
  t = (-dz_hat-sqrt( max(dz_hat^2 - 4*g/2*(z_land-z_hat),0) ))/(-g);
end

== matlab function playback_data_4/Control/Behavior Control/Primary and Lateral Behavior/Closed Loop Compensation/ESTIMATE CLOSED LOOP ERROR Y FOR VARIABLE SPEED ==
  data: dx_land_hist input; A_cl output; delta_ux_hist input; dx_lift_hist input; dx_star_hist input; B_dx_versus_x0 parameter; W_real input; epsilon_0 output; c output; A_cl_nb output; epsilon_0_nb output; c_nb output
function [A_cl, epsilon_0, c, ...
          A_cl_nb, epsilon_0_nb, c_nb] = error_fitting_dxstar...
         (dx_land_hist, delta_ux_hist, dx_lift_hist, dx_star_hist,...
          B_dx_versus_x0, W_real)
% data_length = min([length(dx_lift_hist), filter_length]);
data_length = length(dx_lift_hist);
assert(data_length < 100);
% add fake data
fake_dx_land_err_magnitude = 0.1; fake_dx_star_magnitude = 0.1;
[fgrid_dx_land_err, fgrid_dx_star, fgrid_dx_lift_err] = ...
    meshgrid(fake_dx_land_err_magnitude*[-1 1],fake_dx_star_magnitude*[-1 1],0);
fake_data_length = numel(fgrid_dx_land_err);
fake_dx_land_err = fgrid_dx_land_err(:);
fake_dx_star = fgrid_dx_star(:);
fake_dx_lift_err = fgrid_dx_lift_err(:);
fake_delta_ux = zeros(fake_data_length,1);
% assert(fake_data_length<100);
% assert(filter_length<100);
% fake_dx_land_err = linspace(-0.1, 0.1, fake_data_length)';
% fake_dx_lift_err = zeros(fake_data_length,1);
% fake_delta_ux = zeros(fake_data_length,1);
% fake_dx_star = linspace(-0.25, 0.25, fake_data_length)';
dx_land_err = [reshape(dx_land_hist(1:data_length)-dx_star_hist(1:data_length),...
                       data_length, 1); fake_dx_land_err];
dx_lift_err = [reshape(dx_lift_hist(1:data_length)-dx_star_hist(1:data_length),...
                       data_length, 1); fake_dx_lift_err];
dx_star = [reshape(dx_star_hist(1:data_length), data_length,1); fake_dx_star];
delta_ux = [reshape(delta_ux_hist(1:data_length), data_length, 1); fake_delta_ux];
% weighted least squares
W = diag([W_real*ones(1,data_length), ones(1,fake_data_length)]);
Y = dx_lift_err - B_dx_versus_x0*delta_ux;
X = [dx_land_err, dx_star, ones(data_length+fake_data_length,1)];
% linear regression for s_{i+1}-s0 = A_cl*(s_i-s0) + epsilon_0 + c(s0) + B*delta_u
% solve for Y = X*beta, beta column vector
beta_hat = (X'*W*X)\X'*W*Y;
W_nobias = diag([W_real*ones(1,data_length), 0.001*ones(1,fake_data_length)]);
beta_hat_nobias = (X'*W_nobias*X)\X'*W_nobias*Y;
A_cl = beta_hat(1);
c = beta_hat(2);
epsilon_0 = beta_hat(3);
A_cl_nb = beta_hat_nobias(1);
c_nb = beta_hat_nobias(2);
epsilon_0_nb = beta_hat_nobias(3);

== matlab function playback_data_4/Control/Behavior Control/Primary and Lateral Behavior/Circular Buffer/Buffer ==
  data: data input; buffer output size=recorded_steps; trigger input; buffer_size input
function buffer  = buffer_data(data, trigger, buffer_size)

    persistent buffer_memory
    coder.varsize('buffer_memory',100);
    if isempty(buffer_memory)
        buffer_memory = [];
    end
    
    if trigger
        buffer_memory = [data; buffer_memory];
        if size(buffer_memory, 1) > buffer_size
            buffer_memory = buffer_memory(1:buffer_size,:);
        end
    end
    
    buffer = buffer_memory;

end

== matlab function playback_data_4/Control/Behavior Control/Primary and Lateral Behavior/Circular Buffer/Buffer1 ==
  data: data input; buffer output size=recorded_steps; trigger input; buffer_size input
function buffer  = buffer_data(data, trigger, buffer_size)

    persistent buffer_memory
    coder.varsize('buffer_memory',100);
    if isempty(buffer_memory)
        buffer_memory = [];
    end
    
    if trigger
        buffer_memory = [data; buffer_memory];
        if size(buffer_memory, 1) > buffer_size
            buffer_memory = buffer_memory(1:buffer_size,:);
        end
    end
    
    buffer = buffer_memory;

end
